simulink model "realimentacion"  (R2024a)
settings: Solver=VariableStepAuto  StartTime=0.0  StopTime=10.0  RelTol=1e-3
settings Model: Creator=Perez  LastModifiedBy=Perez

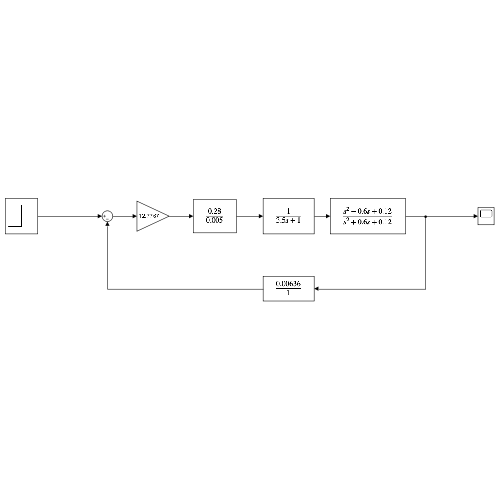
[thumbnail: Simulink's stored preview of the top-level diagram]
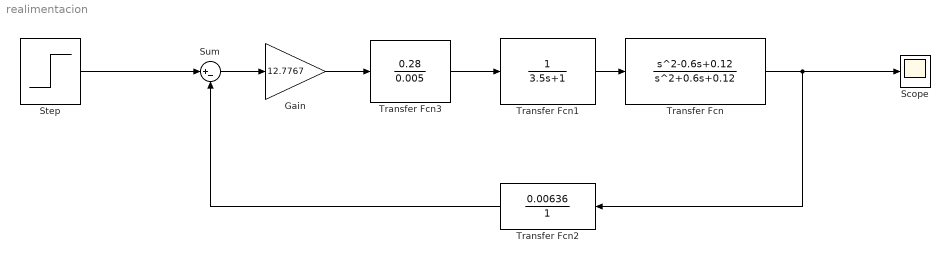
== system realimentacion ==
  Gain : Gain  Gain=12.7767
  Scope : Scope
  Step : Step  SampleTime=0
  Sum : Sum  Inputs=|+-
  Transfer Fcn : TransferFcn  Numerator=[1 -0.6 0.12]  Denominator=[1 0.6 0.12]
  Transfer Fcn1 : TransferFcn  Denominator=[3.5 1]
  Transfer Fcn2 : TransferFcn  Numerator=[0.00636]  Denominator=[1]
  Transfer Fcn3 : TransferFcn  Numerator=[0.28]  Denominator=[0.005]
  wires:
  Transfer Fcn1/1 -> Transfer Fcn/1
  Transfer Fcn/1 -> Scope/1, Transfer Fcn2/1
  Step/1 -> Sum/1
  Transfer Fcn2/1 -> Sum/2
  Sum/1 -> Gain/1
  Gain/1 -> Transfer Fcn3/1
  Transfer Fcn3/1 -> Transfer Fcn1/1
